simulink model "power_thyristor"  (R2014a)
settings: Solver=ode23tb  SolverMode=SingleTasking  StartTime=0.0  StopTime=0.1  RelTol=1e-4
libraries: powerlib x9, powerlib_meascontrol x2
Description:
  | Copyright 2008-2014 The MathWorks, Inc.
settings Model: ExtModeTrigMode=oneshot  ExtModeArmWhenConnect=off  ExtModeAutoUpdateStatusClock=off  Creator=MathWorks  LastModifiedBy=User
settings DataIOCC: LimitDataPoints=off  SignalLoggingSaveFormat=ModelDataLogs  SaveOutput=off  TimeSaveName=t  SignalLoggingName=sigsOut
settings OptimizationCC: BooleanDataType=off  ExpressionDepthLimit=2147483647  InitFltsAndDblsToZero=on  EfficientMapNaN2IntZero=off
settings DebuggingCC: SaveWithParameterizedLinksMsg=none  UnderspecifiedInitializationDetection=Classic  SignalResolutionControl=TryResolveAllWithWarning  SolverPrmCheckMsg=none  MultiTaskDSMMsg=warning  MultiTaskCondExecSysMsg=none  SigSpecEnsureSampleTimeMsg=none  FcnCallInpInsideContextMsg=UseLocalSettings  UnconnectedInputMsg=none  UnconnectedOutputMsg=none  StateNameClashWarn=warning
settings HardwareCC: TargetUnknown=on
settings RTWCC: IncludeERTFirstTime=on
settings GRTTargetCC: TargetFcnLib=ansi_tfl_tmw.mat  CombineOutputUpdateFcns=off  GRTInterface=on

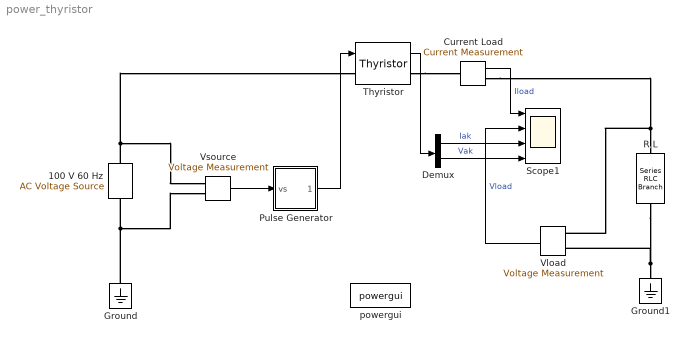
== system power_thyristor ==
  " Pulse Generator" : Subsystem
      mask Display: plot(0,0,100,100,[90,75,75,60,60,35,35,20,20,10],[20,20,80,80,20,20,80,80,20,20])
  100 V 60 Hz : powerlib/Electrical Sources/AC Voltage Source  Description=source block  Amplitude=100  Phase=0  Frequency=60  SampleTime=0  Measurements=None
      settings: AttributesFormatString=\n
  Current Load : powerlib/Measurements/Current Measurement  Tag=PoWeRsYsTeMmEaSuReMeNt  PhasorSimulation=off  OutputType=Magnitude  PSBequivalent=0
  Demux : Demux  Outputs=2
  Ground : powerlib/Elements/Ground  LConnTagsString=a
  Ground1 : powerlib/Elements/Ground  LConnTagsString=a
  R L : powerlib/Elements/Series RLC Branch  LConnTagsString=__new0  RConnTagsString=__new0  BranchType=RL  Resistance=1  Inductance=10e-03  SetiL0=off  InitialCurrent=0  Capacitance=[]  Setx0=off  InitialVoltage=0  Measurements=None
  Scope1 : Scope  NumInputPorts=4
      settings: TimeRange=0.1  YMin=-50~-100~0~-200  YMax=50~100~40~200
  Thyristor : powerlib/Power Electronics/Thyristor  Ron=1e-3  Lon=0  Vf=0.8  IC=0  Rs=20  Cs=4e-6  Measurements=on
      settings: AttributesFormatString=\n
  Vload : powerlib/Measurements/Voltage Measurement  Tag=PoWeRsYsTeMmEaSuReMeNt  PhasorSimulation=off  OutputType=Magnitude  PSBequivalent=0
  Vsource : powerlib/Measurements/Voltage Measurement  Tag=PoWeRsYsTeMmEaSuReMeNt  PhasorSimulation=off  OutputType=Magnitude  PSBequivalent=0
  powergui : powerlib/powergui  SimulationMode=Continuous  SolverType=Tustin  SampleTime=0  frequency=60  SPID=off  DisableSnubberDevices=off  DisableRonSwitches=off  DisableVfSwitches=off  SwTol=0  Interpol=off  DisplayEquations=off  Ts=0  methode=off  frequencyindice=60  Pbase=100e6  ErrMax=1e-4  Iterations=50  UnitsV=kV  UnitsW=MW  FunctionMessages=off  echomessages=off  HookPort=off  EnableUseOfTLC=off  x0status=blocks  RestoreLinks=warning  ResistiveCurrentMeasurement=off  Frange=[0:2:500]  Ylog=off  Xlog=on  ShowGrid=off  save=off  variable=ZData  structure=0  ZoomFFT=on  StartTime=0.0  cycles=1  DisplayStyle=1  fundamental=60  FreqAxis=off  MaxFrequency=1000  frequencyindicesteady=1  RmsSteady=1  display=off
  wires:
  Demux/1 -> Scope1/3  "Iak"
  Demux/2 -> Scope1/4  "Vak"
  Thyristor/1 -> Demux/1
  Current Load/1 -> Scope1/1  "Iload"
  Vload/1 -> Scope1/2  "Vload"
  Vsource/1 -> " Pulse Generator"/1(vs)
  " Pulse Generator"/1(Pulses) -> Thyristor/1
  connections:
  Thyristor/RConn1 -- Current Load/LConn1
  Current Load/RConn1 -- Vload/LConn1 -- R L/LConn1
  Ground1/LConn1 -- R L/RConn1 -- Vload/LConn2
  Ground/LConn1 -- Vsource/LConn2 -- 100 V 60 Hz/LConn1
  100 V 60 Hz/RConn1 -- Vsource/LConn1 -- Thyristor/LConn1

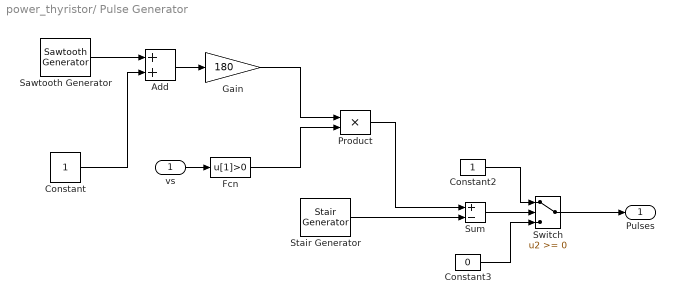
== system power_thyristor/ Pulse Generator ==
  vs : Inport
  Add : Sum
  Constant : Constant
  Constant2 : Constant
  Constant3 : Constant  Value=0
  Fcn : Fcn  Expr=u[1]>0
  Gain : Gain  Gain=180
  Product : Product  SaturateOnIntegerOverflow=on  InputSameDT=on  OutDataTypeStr=Inherit: Same as first input
  Sawtooth Generator : powerlib_meascontrol/Pulse & Signal Generators/Sawtooth Generator  Freq=60  Phase=360  Ts=0
      settings: AttributesFormatString=Freq=%<Freq>\nPhase=%<Phase>
  Stair Generator : powerlib_meascontrol/Pulse & Signal Generators/Stair Generator  t="[ 0  1/60 2/60 3/60 4/60 ]"  e="[20   50   80   110  140  ]"  Ts=0
  Sum : Sum  Inputs=+-  SaturateOnIntegerOverflow=on  InputSameDT=on  OutDataTypeStr=Inherit: Same as first input
  Switch : Switch  SaturateOnIntegerOverflow=on  InputSameDT=on
  Pulses : Outport
  wires:
  Product/1 -> Sum/1
  Fcn/1 -> Product/2
  Constant2/1 -> Switch/1
  Sum/1 -> Switch/2
  Switch/1 -> Pulses/1
  Constant3/1 -> Switch/3
  Stair Generator/1 -> Sum/2
  Sawtooth Generator/1 -> Add/1
  Add/1 -> Gain/1
  Constant/1 -> Add/2
  Gain/1 -> Product/1
  vs/1 -> Fcn/1
